simulink model "LedCircle"  (R2013b)
settings: Solver=FixedStepDiscrete  StartTime=0.0  StopTime=120.0  FixedStep=0.1  MaxStep=0.1  RelTol=1e-3
libraries: ardrone_lib x1
settings Model: Creator=benjamin  LastModifiedBy=Jon Even ROSENGREN
settings OptimizationCC: InitFltsAndDblsToZero=on  OptimizeModelRefInitCode=on  LifeSpan=1
settings RTWCC: SystemTargetFile=ardrone.tlc  TemplateMakefile=ardrone.tmf  Description=AR.Drone_v2  ProcessScript=ardrone_make_rtw_hook  TargetLang=C++
settings CodeAppCC: IgnoreCustomStorageClasses=off
settings STFCustomTargetCC: GenerateSampleERTMain=on  ModelReferenceCompliant=off  CombineOutputUpdateFcns=on  ERTCustomFileBanners=on  SupportContinuousTime=off  SupportNonInlinedSFcns=off  MATLABClassNameForMDSCustomization=Simulink.SoftwareTarget.ERTCustomization  GRTInterface=off  SystemTargetFile=ardrone.tlc
settings ERTTargetCC: CodeReplacementLibrary=ANSI_C  GenerateSampleERTMain=on  ModelReferenceCompliant=off  ParMdlRefBuildCompliant=off  CompOptLevelCompliant=off  ConcurrentExecutionCompliant=off  ERTFirstTimeCompliant=off  ModelStepFunctionPrototypeControlCompliant=off  CPPClassGenCompliant=off  ERTSrcFileBannerTemplate=example_banner.tlc  ERTHdrFileBannerTemplate=example_banner.tlc  ERTCustomFileTemplate=ardrone_file_process.tlc

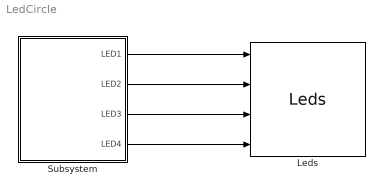
== system LedCircle ==
  Leds : ardrone_lib/Leds  SystemSampleTime=-1
  Subsystem : Subsystem
  wires:
  Subsystem/2(LED2) -> Leds/2
  Subsystem/1(LED1) -> Leds/1
  Subsystem/3(LED3) -> Leds/3
  Subsystem/4(LED4) -> Leds/4

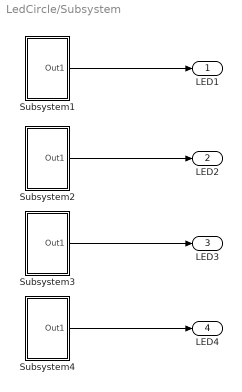
== system LedCircle/Subsystem ==
  Subsystem1 : Subsystem
  Subsystem2 : Subsystem
  Subsystem3 : Subsystem
  Subsystem4 : Subsystem
  LED1 : Outport
  LED2 : Outport  Port=2
  LED3 : Outport  Port=3
  LED4 : Outport  Port=4
  wires:
  Subsystem4/1(Out1) -> LED4/1
  Subsystem3/1(Out1) -> LED3/1
  Subsystem2/1(Out1) -> LED2/1
  Subsystem1/1(Out1) -> LED1/1

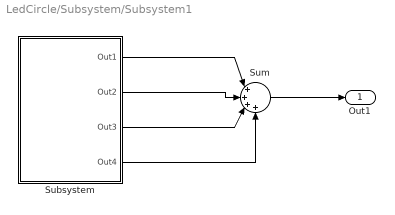
== system LedCircle/Subsystem/Subsystem1 ==
  Subsystem : Subsystem
  Sum : Sum  Inputs=|++++
  Out1 : Outport
  wires:
  Subsystem/2(Out2) -> Sum/2
  Subsystem/1(Out1) -> Sum/1
  Sum/1 -> Out1/1
  Subsystem/3(Out3) -> Sum/3
  Subsystem/4(Out4) -> Sum/4

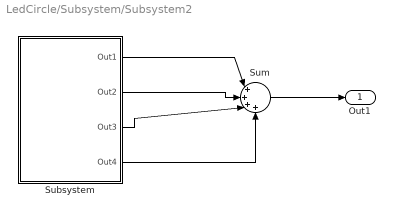
== system LedCircle/Subsystem/Subsystem2 ==
  Subsystem : Subsystem
  Sum : Sum  Inputs=|++++
  Out1 : Outport
  wires:
  Subsystem/2(Out2) -> Sum/2
  Subsystem/1(Out1) -> Sum/1
  Sum/1 -> Out1/1
  Subsystem/3(Out3) -> Sum/3
  Subsystem/4(Out4) -> Sum/4

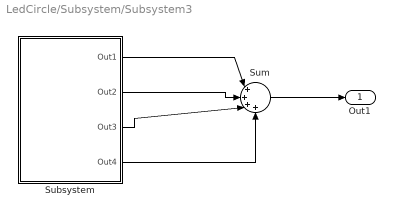
== system LedCircle/Subsystem/Subsystem3 ==
  Subsystem : Subsystem
  Sum : Sum  Inputs=|++++
  Out1 : Outport
  wires:
  Subsystem/2(Out2) -> Sum/2
  Subsystem/1(Out1) -> Sum/1
  Sum/1 -> Out1/1
  Subsystem/3(Out3) -> Sum/3
  Subsystem/4(Out4) -> Sum/4

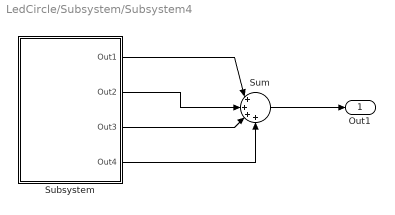
== system LedCircle/Subsystem/Subsystem4 ==
  Subsystem : Subsystem
  Sum : Sum  Inputs=|++++
  Out1 : Outport
  wires:
  Subsystem/2(Out2) -> Sum/2
  Subsystem/1(Out1) -> Sum/1
  Sum/1 -> Out1/1
  Subsystem/3(Out3) -> Sum/3
  Subsystem/4(Out4) -> Sum/4

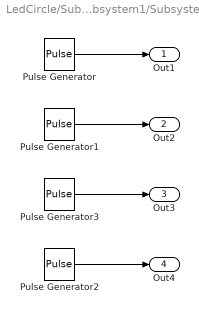
== system LedCircle/Subsystem/Subsystem1/Subsystem ==
  Pulse Generator : DiscretePulseGenerator  PulseType=Time based  Amplitude=0  Period=4  PulseWidth=25
  Pulse Generator1 : DiscretePulseGenerator  PulseType=Time based  Period=4  PulseWidth=25  PhaseDelay=1
  Pulse Generator2 : DiscretePulseGenerator  PulseType=Time based  Amplitude=3  Period=4  PulseWidth=25  PhaseDelay=3
  Pulse Generator3 : DiscretePulseGenerator  PulseType=Time based  Amplitude=2  Period=4  PulseWidth=25  PhaseDelay=2
  Out1 : Outport
  Out2 : Outport  Port=2
  Out3 : Outport  Port=3
  Out4 : Outport  Port=4
  wires:
  Pulse Generator3/1 -> Out3/1
  Pulse Generator1/1 -> Out2/1
  Pulse Generator2/1 -> Out4/1
  Pulse Generator/1 -> Out1/1

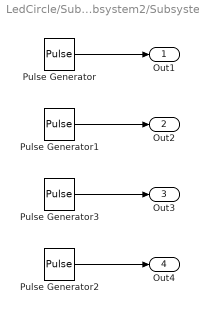
== system LedCircle/Subsystem/Subsystem2/Subsystem ==
  Pulse Generator : DiscretePulseGenerator  PulseType=Time based  Period=4  PulseWidth=25
  Pulse Generator1 : DiscretePulseGenerator  PulseType=Time based  Amplitude=2  Period=4  PulseWidth=25  PhaseDelay=1
  Pulse Generator2 : DiscretePulseGenerator  PulseType=Time based  Amplitude=0  Period=4  PulseWidth=25  PhaseDelay=3
  Pulse Generator3 : DiscretePulseGenerator  PulseType=Time based  Amplitude=3  Period=4  PulseWidth=25  PhaseDelay=2
  Out1 : Outport
  Out2 : Outport  Port=2
  Out3 : Outport  Port=3
  Out4 : Outport  Port=4
  wires:
  Pulse Generator3/1 -> Out3/1
  Pulse Generator1/1 -> Out2/1
  Pulse Generator2/1 -> Out4/1
  Pulse Generator/1 -> Out1/1

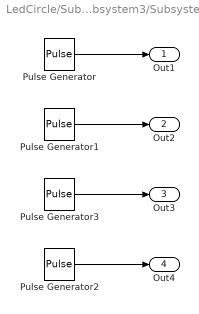
== system LedCircle/Subsystem/Subsystem3/Subsystem ==
  Pulse Generator : DiscretePulseGenerator  PulseType=Time based  Amplitude=2  Period=4  PulseWidth=25
  Pulse Generator1 : DiscretePulseGenerator  PulseType=Time based  Amplitude=3  Period=4  PulseWidth=25  PhaseDelay=1
  Pulse Generator2 : DiscretePulseGenerator  PulseType=Time based  Period=4  PulseWidth=25  PhaseDelay=3
  Pulse Generator3 : DiscretePulseGenerator  PulseType=Time based  Amplitude=0  Period=4  PulseWidth=25  PhaseDelay=2
  Out1 : Outport
  Out2 : Outport  Port=2
  Out3 : Outport  Port=3
  Out4 : Outport  Port=4
  wires:
  Pulse Generator3/1 -> Out3/1
  Pulse Generator1/1 -> Out2/1
  Pulse Generator2/1 -> Out4/1
  Pulse Generator/1 -> Out1/1

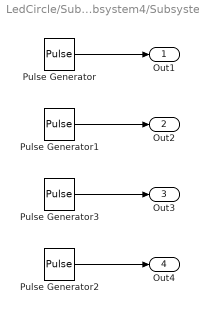
== system LedCircle/Subsystem/Subsystem4/Subsystem ==
  Pulse Generator : DiscretePulseGenerator  PulseType=Time based  Amplitude=3  Period=4  PulseWidth=25
  Pulse Generator1 : DiscretePulseGenerator  PulseType=Time based  Amplitude=0  Period=4  PulseWidth=25  PhaseDelay=1
  Pulse Generator2 : DiscretePulseGenerator  PulseType=Time based  Amplitude=2  Period=4  PulseWidth=25  PhaseDelay=3
  Pulse Generator3 : DiscretePulseGenerator  PulseType=Time based  Period=4  PulseWidth=25  PhaseDelay=2
  Out1 : Outport
  Out2 : Outport  Port=2
  Out3 : Outport  Port=3
  Out4 : Outport  Port=4
  wires:
  Pulse Generator3/1 -> Out3/1
  Pulse Generator1/1 -> Out2/1
  Pulse Generator2/1 -> Out4/1
  Pulse Generator/1 -> Out1/1
